simulink model "Hardmon"  (R2025b)
settings: Solver=ode8  StartTime=0.0  StopTime=10  FixedStep=0.0001  RelTol=1e-3
undefined symbols (not defined in the file): BMS_Contactor_Command
settings Model: DataDictionary=rev3_data.sldd  Creator=heyka  LastModifiedBy=diego
settings DataIOCC: ExternalInput=test_temp.getElement('Temp 1'),test_temp.getElement('Temp 2')  LoadExternalInput=on
settings OptimizationCC: DefaultParameterBehavior=Inlined  EnhancedBackFolding=on  PassReuseOutputArgsThreshold=0.0  ZeroExternalMemoryAtStartup=off  ZeroInternalMemoryAtStartup=off  OptimizeBlockOrder=speed  DifferentSizesBufferReuse=on  OptimizationCustomize=off
settings DebuggingCC: SolverPrmCheckMsg=warning  ParameterTunabilityLossMsg=error  StateNameClashWarn=warning
settings HardwareCC: ProdBitPerInt=16.0  ProdBitPerPointer=16.0  ProdBitPerSizeT=16.0  ProdBitPerPtrDiffT=16.0  ProdLargestAtomicFloat=None  ProdWordSize=16.0  ProdHWDeviceType=STMicroelectronics->ST10/Super10
settings SFSimCC: MATLABDynamicMemAlloc=off  SimTargetLang=C++  SimDLTargetLibrary=mkl-dnn
settings RTWCC: GenCodeOnly=on  Toolchain=MinGW64 | gmake (64-bit Windows)  BuildConfiguration=Faster Runs  TargetLang=C++  GPUComputeCapability=3.5
settings CodeAppCC: ForceParamTrailComments=on  OperatorAnnotations=on  StateflowObjectComments=on
settings GRTTargetCC: TargetLangStandard=C++11 (ISO)  CodeInterfacePackaging=C++ class  SubcomponentCodeInterfacePackaging=C++ class

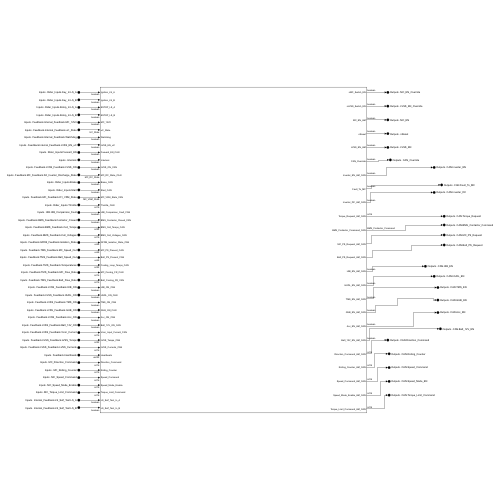
[thumbnail: Simulink's stored preview of the top-level diagram]
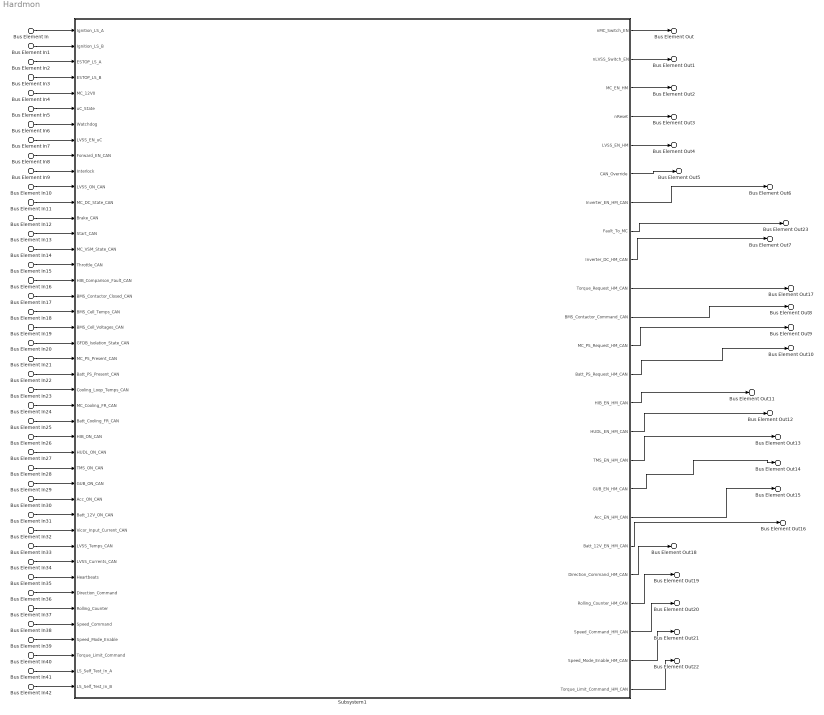
== system Hardmon ==
  Bus Element In2 : Inport  PortName=Inputs  Element=Rider_Inputs.Estop_In.LS_A
  Bus Element In3 : Inport  PortName=Inputs  Element=Rider_Inputs.Estop_In.LS_B
  Bus Element In1 : Inport  PortName=Inputs  Element=Rider_Inputs.Key_In.LS_B
  Bus Element In : Inport  PortName=Inputs  Element=Rider_Inputs.Key_In.LS_A
  Bus Element In8 : Inport  PortName=Inputs  Element=Rider_Inputs.Forward_EN
  Bus Element In12 : Inport  PortName=Inputs  Element=Rider_Inputs.Brake
  Bus Element In13 : Inport  PortName=Inputs  Element=Rider_Inputs.Start
  Bus Element In15 : Inport  PortName=Inputs  Element=Rider_Inputs.Throttle
  Bus Element In4 : Inport  PortName=Inputs  Element=Feedback.Internal_Feedback.MC_12V0
  Bus Element In5 : Inport  PortName=Inputs  Element=Feedback.Internal_Feedback.uC_State
  Bus Element In6 : Inport  PortName=Inputs  Element=Feedback.Internal_Feedback.Watchdog
  Bus Element In7 : Inport  PortName=Inputs  Element=Feedback.Internal_Feedback.LVSS_EN_uC
  Bus Element In10 : Inport  PortName=Inputs  Element=Feedback.LVSS_Feedback.LVSS_ON
  Bus Element In26 : Inport  PortName=Inputs  Element=Feedback.LVSS_Feedback.HIB_ON
  Bus Element In27 : Inport  PortName=Inputs  Element=Feedback.LVSS_Feedback.HUDL_ON
  Bus Element In28 : Inport  PortName=Inputs  Element=Feedback.LVSS_Feedback.TMS_ON
  Bus Element In29 : Inport  PortName=Inputs  Element=Feedback.LVSS_Feedback.GUB_ON
  Bus Element In30 : Inport  PortName=Inputs  Element=Feedback.LVSS_Feedback.Acc_ON
  Bus Element In31 : Inport  PortName=Inputs  Element=Feedback.LVSS_Feedback.Batt_12V_ON
  Bus Element In32 : Inport  PortName=Inputs  Element=Feedback.LVSS_Feedback.Vicor_Current
  Bus Element In33 : Inport  PortName=Inputs  Element=Feedback.LVSS_Feedback.LVSS_Temps
  Bus Element In34 : Inport  PortName=Inputs  Element=Feedback.LVSS_Feedback.LVSS_Currents
  Bus Element In11 : Inport  PortName=Inputs  Element=Feedback.MC_Feedback.D4_Inverter_Discharge_State
  Bus Element In14 : Inport  PortName=Inputs  Element=Feedback.MC_Feedback.D1_VSM_State
  Bus Element In17 : Inport  PortName=Inputs  Element=Feedback.BMS_Feedback.Contactor_Closed
  Bus Element In18 : Inport  PortName=Inputs  Element=Feedback.BMS_Feedback.Cell_Temps
  Bus Element In19 : Inport  PortName=Inputs  Element=Feedback.BMS_Feedback.Cell_Voltages
  Bus Element In20 : Inport  PortName=Inputs  Element=Feedback.GFDB_Feedback.Isolation_State
  Bus Element In21 : Inport  PortName=Inputs  Element=Feedback.TMS_Feedback.MC_Speed_Out
  Bus Element In22 : Inport  PortName=Inputs  Element=Feedback.TMS_Feedback.Batt_Speed_Out
  Bus Element In23 : Inport  PortName=Inputs  Element=Feedback.TMS_Feedback.Temperatures
  Bus Element In24 : Inport  PortName=Inputs  Element=Feedback.TMS_Feedback.MC_Flow_Rate
  Bus Element In25 : Inport  PortName=Inputs  Element=Feedback.TMS_Feedback.Batt_Flow_Rate
  Bus Element In35 : Inport  PortName=Inputs  Element=Feedback.Heartbeats
  Bus Element In9 : Inport  PortName=Inputs  Element=Interlock
  Bus Element In16 : Inport  PortName=Inputs  Element=HIB.HIB_Comparison_Fault
  Bus Element In36 : Inport  PortName=Inputs  Element=MC_Direction_Command
  Bus Element In37 : Inport  PortName=Inputs  Element=MC_Rolling_Counter
  Bus Element In38 : Inport  PortName=Inputs  Element=MC_Speed_Command
  Bus Element In39 : Inport  PortName=Inputs  Element=MC_Speed_Mode_Enable
  Bus Element In40 : Inport  PortName=Inputs  Element=MC_Torque_Limit_Command
  Bus Element In41 : Inport  PortName=Inputs  Element=Internal_Feedback.LS_Self_Test.LS_A
  Bus Element In42 : Inport  PortName=Inputs  Element=Internal_Feedback.LS_Self_Test.LS_B
  Subsystem1 : Subsystem
  Bus Element Out : Outport  PortName=Outputs  Element=MC_EN_Override
  Bus Element Out1 : Outport  PortName=Outputs  Element=LVSS_EN_Override
  Bus Element Out2 : Outport  PortName=Outputs  Element=MC_EN
  Bus Element Out3 : Outport  PortName=Outputs  Element=nReset
  Bus Element Out4 : Outport  PortName=Outputs  Element=LVSS_EN
  Bus Element Out5 : Outport  PortName=Outputs  Element=CAN_Override
  Bus Element Out6 : Outport  PortName=Outputs  Element=CAN.Inverter_EN
  Bus Element Out23 : Outport  PortName=Outputs  Element=CAN.Fault_To_MC
  Bus Element Out7 : Outport  PortName=Outputs  Element=CAN.Inverter_DC
  Bus Element Out17 : Outport  PortName=Outputs  Element=CAN.Torque_Request
  Bus Element Out8 : Outport  PortName=Outputs  Element=CAN.BMS_Contactor_Command
  Bus Element Out9 : Outport  PortName=Outputs  Element=CAN.MC_PS_Request
  Bus Element Out10 : Outport  PortName=Outputs  Element=CAN.Batt_PS_Request
  Bus Element Out11 : Outport  PortName=Outputs  Element=CAN.HIB_EN
  Bus Element Out12 : Outport  PortName=Outputs  Element=CAN.HUDL_EN
  Bus Element Out13 : Outport  PortName=Outputs  Element=CAN.TMS_EN
  Bus Element Out14 : Outport  PortName=Outputs  Element=CAN.GUB_EN
  Bus Element Out15 : Outport  PortName=Outputs  Element=CAN.Acc_EN
  Bus Element Out16 : Outport  PortName=Outputs  Element=CAN.Batt_12V_EN
  Bus Element Out18 : Outport  PortName=Outputs  Element=CAN.Direction_Command
  Bus Element Out19 : Outport  PortName=Outputs  Element=CAN.Rolling_Counter
  Bus Element Out20 : Outport  PortName=Outputs  Element=CAN.Speed_Command
  Bus Element Out21 : Outport  PortName=Outputs  Element=CAN.Speed_Mode_EN
  Bus Element Out22 : Outport  PortName=Outputs  Element=CAN.Torque_Limit_Command
  wires:
  Bus Element In/1 -> Subsystem1/1(Ignition_LS_A)
  Bus Element In1/1 -> Subsystem1/2(Ignition_LS_B)
  Bus Element In2/1 -> Subsystem1/3(ESTOP_LS_A)
  Bus Element In3/1 -> Subsystem1/4(ESTOP_LS_B)
  Bus Element In4/1 -> Subsystem1/5(MC_12V0)
  Bus Element In5/1 -> Subsystem1/6(uC_State)
  Bus Element In6/1 -> Subsystem1/7(Watchdog)
  Bus Element In7/1 -> Subsystem1/8(LVSS_EN_uC)
  Bus Element In8/1 -> Subsystem1/9(Forward_EN_CAN)
  Bus Element In9/1 -> Subsystem1/10(Interlock)
  Bus Element In10/1 -> Subsystem1/11(LVSS_ON_CAN)
  Bus Element In11/1 -> Subsystem1/12(MC_DC_State_CAN)
  Bus Element In12/1 -> Subsystem1/13(Brake_CAN)
  Bus Element In13/1 -> Subsystem1/14(Start_CAN)
  Bus Element In14/1 -> Subsystem1/15(MC_VSM_State_CAN)
  Bus Element In15/1 -> Subsystem1/16(Throttle_CAN)
  Bus Element In16/1 -> Subsystem1/17(HIB_Comparison_Fault_CAN)
  Bus Element In17/1 -> Subsystem1/18(BMS_Contactor_Closed_CAN)
  Bus Element In18/1 -> Subsystem1/19(BMS_Cell_Temps_CAN)
  Bus Element In19/1 -> Subsystem1/20(BMS_Cell_Voltages_CAN)
  Bus Element In20/1 -> Subsystem1/21(GFDB_Isolation_State_CAN)
  Bus Element In21/1 -> Subsystem1/22(MC_PS_Present_CAN)
  Bus Element In22/1 -> Subsystem1/23(Batt_PS_Present_CAN)
  Bus Element In23/1 -> Subsystem1/24(Cooling_Loop_Temps_CAN)
  Bus Element In24/1 -> Subsystem1/25(MC_Cooling_FR_CAN)
  Bus Element In25/1 -> Subsystem1/26(Batt_Cooling_FR_CAN)
  Bus Element In26/1 -> Subsystem1/27(HIB_ON_CAN)
  Bus Element In27/1 -> Subsystem1/28(HUDL_ON_CAN)
  Bus Element In28/1 -> Subsystem1/29(TMS_ON_CAN)
  Bus Element In29/1 -> Subsystem1/30(GUB_ON_CAN)
  Bus Element In30/1 -> Subsystem1/31(Acc_ON_CAN)
  Bus Element In31/1 -> Subsystem1/32(Batt_12V_ON_CAN)
  Bus Element In32/1 -> Subsystem1/33(Vicor_Input_Current_CAN)
  Bus Element In33/1 -> Subsystem1/34(LVSS_Temps_CAN)
  Bus Element In34/1 -> Subsystem1/35(LVSS_Currents_CAN)
  Bus Element In35/1 -> Subsystem1/36(Heartbeats)
  Bus Element In36/1 -> Subsystem1/37(Direction_Command)
  Bus Element In37/1 -> Subsystem1/38(Rolling_Counter)
  Bus Element In38/1 -> Subsystem1/39(Speed_Command)
  Bus Element In39/1 -> Subsystem1/40(Speed_Mode_Enable)
  Bus Element In40/1 -> Subsystem1/41(Torque_Limit_Command)
  Bus Element In41/1 -> Subsystem1/42(LS_Self_Test_In_A)
  Bus Element In42/1 -> Subsystem1/43(LS_Self_Test_In_B)
  Subsystem1/1(nMC_Switch_EN) -> Bus Element Out/1
  Subsystem1/2(nLVSS_Switch_EN) -> Bus Element Out1/1
  Subsystem1/3(MC_EN_HM) -> Bus Element Out2/1
  Subsystem1/4(nReset) -> Bus Element Out3/1
  Subsystem1/5(LVSS_EN_HM) -> Bus Element Out4/1
  Subsystem1/6(CAN_Override) -> Bus Element Out5/1
  Subsystem1/7(Inverter_EN_HM_CAN) -> Bus Element Out6/1
  Subsystem1/9(Inverter_DC_HM_CAN) -> Bus Element Out7/1
  Subsystem1/11(BMS_Contactor_Command_CAN) -> Bus Element Out8/1
  Subsystem1/12(MC_PS_Request_HM_CAN) -> Bus Element Out9/1
  Subsystem1/13(Batt_PS_Request_HM_CAN) -> Bus Element Out10/1
  Subsystem1/14(HIB_EN_HM_CAN) -> Bus Element Out11/1
  Subsystem1/15(HUDL_EN_HM_CAN) -> Bus Element Out12/1
  Subsystem1/16(TMS_EN_HM_CAN) -> Bus Element Out13/1
  Subsystem1/17(GUB_EN_HM_CAN) -> Bus Element Out14/1
  Subsystem1/18(Acc_EN_HM_CAN) -> Bus Element Out15/1
  Subsystem1/19(Batt_12V_EN_HM_CAN) -> Bus Element Out16/1
  Subsystem1/10(Torque_Request_HM_CAN) -> Bus Element Out17/1
  Subsystem1/20(Direction_Command_HM_CAN) -> Bus Element Out18/1
  Subsystem1/21(Rolling_Counter_HM_CAN) -> Bus Element Out19/1
  Subsystem1/22(Speed_Command_HM_CAN) -> Bus Element Out20/1
  Subsystem1/23(Speed_Mode_Enable_HM_CAN) -> Bus Element Out21/1
  Subsystem1/24(Torque_Limit_Command_HM_CAN) -> Bus Element Out22/1
  Subsystem1/8(Fault_To_MC) -> Bus Element Out23/1

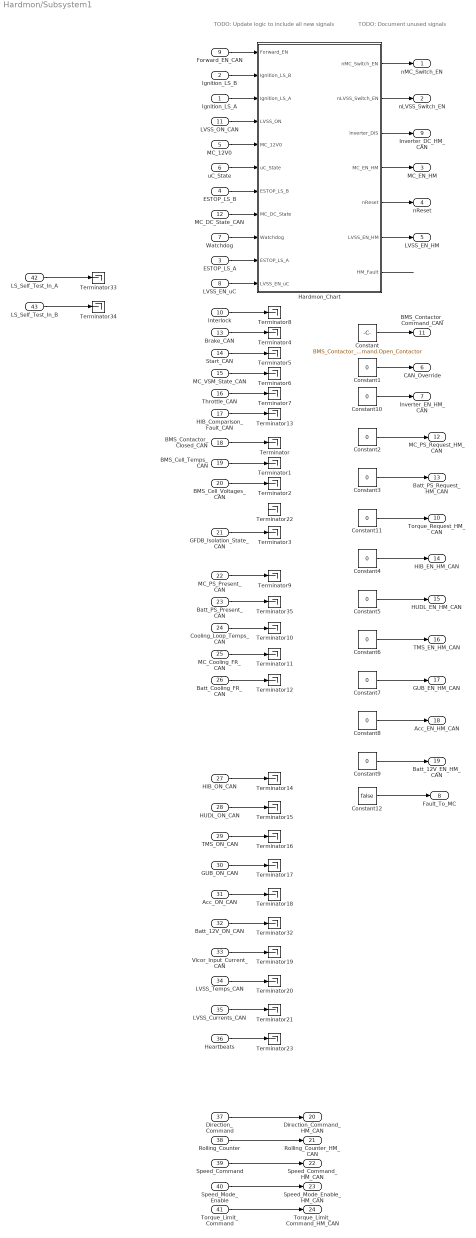
== system Hardmon/Subsystem1 ==
  note: TODO: Update logic to include all new signals
  note: TODO: Document unused signals
  Ignition_LS_A : Inport  OutDataTypeStr=boolean
  Ignition_LS_B : Inport  Port=2  OutDataTypeStr=boolean
  ESTOP_LS_A : Inport  Port=3  OutDataTypeStr=boolean
  ESTOP_LS_B : Inport  Port=4  OutDataTypeStr=boolean
  MC_12V0 : Inport  Port=5  OutDataTypeStr=boolean
  uC_State : Inport  Port=6  OutDataTypeStr=Enum: UC_State
  Watchdog : Inport  Port=7  OutDataTypeStr=boolean
  LVSS_EN_uC : Inport  Port=8  OutDataTypeStr=boolean
  Forward_EN_CAN : Inport  Port=9  OutDataTypeStr=boolean
  Interlock : Inport  Port=10  OutDataTypeStr=boolean
  LVSS_ON_CAN : Inport  Port=11  OutDataTypeStr=boolean
  MC_DC_State_CAN : Inport  Port=12  OutDataTypeStr=Enum: MC_DC_State
  Brake_CAN : Inport  Port=13  OutDataTypeStr=boolean
  Start_CAN : Inport  Port=14  OutDataTypeStr=boolean
  MC_VSM_State_CAN : Inport  Port=15  OutDataTypeStr=Enum: MC_VSM_State
  Throttle_CAN : Inport  Port=16  OutDataTypeStr=int16
  HIB_Comparison_Fault_CAN : Inport  Port=17  OutDataTypeStr=boolean
  BMS_Contactor_Closed_CAN : Inport  Port=18  OutDataTypeStr=boolean
  BMS_Cell_Temps_CAN : Inport  Port=19  OutDataTypeStr=int32  PortDimensions=[1,45]
  BMS_Cell_Voltages_CAN : Inport  Port=20  OutDataTypeStr=int16  PortDimensions=[1,100]
  GFDB_Isolation_State_CAN : Inport  Port=21  OutDataTypeStr=uint8
  MC_PS_Present_CAN : Inport  Port=22  OutDataTypeStr=uint8
  Batt_PS_Present_CAN : Inport  Port=23  OutDataTypeStr=uint8
  Cooling_Loop_Temps_CAN : Inport  Port=24  OutDataTypeStr=int32  PortDimensions=[1,5]
  MC_Cooling_FR_CAN : Inport  Port=25  OutDataTypeStr=int16
  Batt_Cooling_FR_CAN : Inport  Port=26  OutDataTypeStr=int16
  HIB_ON_CAN : Inport  Port=27  OutDataTypeStr=boolean
  HUDL_ON_CAN : Inport  Port=28  OutDataTypeStr=boolean
  TMS_ON_CAN : Inport  Port=29  OutDataTypeStr=boolean
  GUB_ON_CAN : Inport  Port=30  OutDataTypeStr=boolean
  Acc_ON_CAN : Inport  Port=31  OutDataTypeStr=boolean
  Batt_12V_ON_CAN : Inport  Port=32  OutDataTypeStr=boolean
  Vicor_Input_Current_CAN : Inport  Port=33  OutDataTypeStr=int16
  LVSS_Temps_CAN : Inport  Port=34  OutDataTypeStr=int32  PortDimensions=[1,6]
  LVSS_Currents_CAN : Inport  Port=35  OutDataTypeStr=int16  PortDimensions=[1,6]
  Heartbeats : Inport  Port=36  OutDataTypeStr=uint32  PortDimensions=[1,5]
  Direction_Command : Inport  Port=37  OutDataTypeStr=int16
  Rolling_Counter : Inport  Port=38  OutDataTypeStr=int16
  Speed_Command : Inport  Port=39  OutDataTypeStr=int16
  Speed_Mode_Enable : Inport  Port=40  OutDataTypeStr=int16
  Torque_Limit_Command : Inport  Port=41  OutDataTypeStr=int16
  LS_Self_Test_In_A : Inport  Port=42  OutDataTypeStr=boolean
  LS_Self_Test_In_B : Inport  Port=43  OutDataTypeStr=boolean
  Constant : Constant  Value=BMS_Contactor_Command.Open_Contactor  OutDataTypeStr=Enum: BMS_Contactor_Command
  Constant{1,4..10} (8 alike) : Constant  Value=0  OutDataTypeStr=boolean
  Constant11 : Constant  Value=0  OutDataTypeStr=int16
  Constant12 : Constant  Value=false  OutDataTypeStr=boolean
  Constant2 : Constant  Value=0  OutDataTypeStr=uint8
  Constant3 : Constant  Value=0  OutDataTypeStr=uint8
  Hardmon_Chart : Stateflow chart  TreatAsAtomicUnit=on
      settings: PortSchema="{\"entries\":[{\"content\":{\"sides\":[{\"content\":{\"connectorIds\":[\"In1\",\"In2\",\"In3\",\"In4\",\"In5\",\"In6\",\"In7\",\"In8\",\"In9\",\"In10\",\"In11\"]},\"type\":\"ConnectorPlacement.EquallySpacedRectSide\",\"uuid\":\"6d1a41ef-67e8-41d6-9adb-1761831f6d0e\"},{\"content\":{\"connectorIds\":[\"Out1\",\"Out7\",\"Out2\",\"Out3\",\"Out4\",\"Out5\",\"Out6\"],\"side\":\"RIGHT\"},\"type\":\"ConnectorPlacement.EquallySpacedRectSide\",\"uuid\":\"1c1f5b1f-9a19-48ee-ac61-8a13c1cfd4a8\"},{\"content\":{\"side\":\"TOP\"},\"type\":\"ConnectorPlacement.EquallySpacedRectSide\",\"uuid\":\"7f8ec887-50f7-4fb3-9eed-5aef04cf2afb\"}]},\"type\":\"ConnectorPlacement.EquallySpacedConnector\",\"uuid\":\"822c8876-1e52-4482-83f3-7114ae95ed93\"}],\"packageUris\":[\"http://schema.mathworks.com/mf0/Connector/R2020b\"],\"version\":\"1.0\"}"
  Terminator{,1..23,32..35} (28 alike) : Terminator
  nMC_Switch_EN : Outport  OutDataTypeStr=boolean
  nLVSS_Switch_EN : Outport  Port=2  OutDataTypeStr=boolean
  MC_EN_HM : Outport  Port=3  OutDataTypeStr=boolean
  nReset : Outport  Port=4  OutDataTypeStr=boolean
  LVSS_EN_HM : Outport  Port=5  OutDataTypeStr=boolean
  CAN_Override : Outport  Port=6  OutDataTypeStr=boolean
  Inverter_EN_HM_CAN : Outport  Port=7  OutDataTypeStr=boolean
  Fault_To_MC : Outport  Port=8  OutDataTypeStr=boolean
  Inverter_DC_HM_CAN : Outport  Port=9  OutDataTypeStr=boolean
  Torque_Request_HM_CAN : Outport  Port=10  OutDataTypeStr=int16
  BMS_Contactor_Command_CAN : Outport  Port=11  OutDataTypeStr=Enum: BMS_Contactor_Command
  MC_PS_Request_HM_CAN : Outport  Port=12
  Batt_PS_Request_HM_CAN : Outport  Port=13
  HIB_EN_HM_CAN : Outport  Port=14  OutDataTypeStr=boolean
  HUDL_EN_HM_CAN : Outport  Port=15  OutDataTypeStr=boolean
  TMS_EN_HM_CAN : Outport  Port=16  OutDataTypeStr=boolean
  GUB_EN_HM_CAN : Outport  Port=17  OutDataTypeStr=boolean
  Acc_EN_HM_CAN : Outport  Port=18  OutDataTypeStr=boolean
  Batt_12V_EN_HM_CAN : Outport  Port=19  OutDataTypeStr=boolean
  Direction_Command_HM_CAN : Outport  Port=20  OutDataTypeStr=int16
  Rolling_Counter_HM_CAN : Outport  Port=21  OutDataTypeStr=int16
  Speed_Command_HM_CAN : Outport  Port=22  OutDataTypeStr=int16
  Speed_Mode_Enable_HM_CAN : Outport  Port=23  OutDataTypeStr=int16
  Torque_Limit_Command_HM_CAN : Outport  Port=24  OutDataTypeStr=int16
  wires:
  Vicor_Input_Current_CAN/1 -> Terminator19/1
  LVSS_Temps_CAN/1 -> Terminator20/1
  MC_PS_Present_CAN/1 -> Terminator9/1
  Torque_Limit_Command/1 -> Torque_Limit_Command_HM_CAN/1
  Heartbeats/1 -> Terminator23/1
  Throttle_CAN/1 -> Terminator7/1
  ? -> Terminator22/1
  BMS_Cell_Temps_CAN/1 -> Terminator1/1
  Hardmon_Chart/1(nMC_Switch_EN) -> nMC_Switch_EN/1
  HIB_ON_CAN/1 -> Terminator14/1
  Constant9/1 -> Batt_12V_EN_HM_CAN/1
  LVSS_Currents_CAN/1 -> Terminator21/1
  Constant11/1 -> Torque_Request_HM_CAN/1
  Rolling_Counter/1 -> Rolling_Counter_HM_CAN/1
  BMS_Cell_Voltages_CAN/1 -> Terminator2/1
  MC_12V0/1 -> Hardmon_Chart/5(MC_12V0)
  GUB_ON_CAN/1 -> Terminator17/1
  Direction_Command/1 -> Direction_Command_HM_CAN/1
  HUDL_ON_CAN/1 -> Terminator15/1
  MC_DC_State_CAN/1 -> Hardmon_Chart/8(MC_DC_State)
  Hardmon_Chart/4(nReset) -> nReset/1
  LVSS_EN_uC/1 -> Hardmon_Chart/11(LVSS_EN_uC)
  Constant7/1 -> GUB_EN_HM_CAN/1
  Constant10/1 -> Inverter_EN_HM_CAN/1
  LVSS_ON_CAN/1 -> Hardmon_Chart/4(LVSS_ON)
  Speed_Mode_Enable/1 -> Speed_Mode_Enable_HM_CAN/1
  Ignition_LS_A/1 -> Hardmon_Chart/3(Ignition_LS_A)
  MC_Cooling_FR_CAN/1 -> Terminator11/1
  ESTOP_LS_A/1 -> Hardmon_Chart/10(ESTOP_LS_A)
  Constant8/1 -> Acc_EN_HM_CAN/1
  ESTOP_LS_B/1 -> Hardmon_Chart/7(ESTOP_LS_B)
  MC_VSM_State_CAN/1 -> Terminator6/1
  Constant/1 -> BMS_Contactor_Command_CAN/1
  Batt_PS_Present_CAN/1 -> Terminator35/1
  Forward_EN_CAN/1 -> Hardmon_Chart/1(Forward_EN)
  TMS_ON_CAN/1 -> Terminator16/1
  Brake_CAN/1 -> Terminator4/1
  Batt_Cooling_FR_CAN/1 -> Terminator12/1
  HIB_Comparison_Fault_CAN/1 -> Terminator13/1
  BMS_Contactor_Closed_CAN/1 -> Terminator/1
  Constant6/1 -> TMS_EN_HM_CAN/1
  Constant4/1 -> HIB_EN_HM_CAN/1
  Hardmon_Chart/7(nLVSS_Switch_EN) -> nLVSS_Switch_EN/1
  Hardmon_Chart/2(Inverter_DIS) -> Inverter_DC_HM_CAN/1
  LS_Self_Test_In_A/1 -> Terminator33/1
  Batt_12V_ON_CAN/1 -> Terminator32/1
  Constant3/1 -> Batt_PS_Request_HM_CAN/1
  Constant2/1 -> MC_PS_Request_HM_CAN/1
  Cooling_Loop_Temps_CAN/1 -> Terminator10/1
  GFDB_Isolation_State_CAN/1 -> Terminator3/1
  Speed_Command/1 -> Speed_Command_HM_CAN/1
  Start_CAN/1 -> Terminator5/1
  LS_Self_Test_In_B/1 -> Terminator34/1
  Hardmon_Chart/5(LVSS_EN_HM) -> LVSS_EN_HM/1
  Hardmon_Chart/3(MC_EN_HM) -> MC_EN_HM/1
  Constant5/1 -> HUDL_EN_HM_CAN/1
  Ignition_LS_B/1 -> Hardmon_Chart/2(Ignition_LS_B)
  Hardmon_Chart/6(HM_Fault) -> ?
  uC_State/1 -> Hardmon_Chart/6(uC_State)
  Acc_ON_CAN/1 -> Terminator18/1
  Watchdog/1 -> Hardmon_Chart/9(Watchdog)
  Constant1/1 -> CAN_Override/1
  Interlock/1 -> Terminator8/1
  Constant12/1 -> Fault_To_MC/1

== stateflow chart Hardmon/Subsystem1/Hardmon_Chart ==
  note: General Notes:
      | - LVSS_EN_HM = LVSS_EN_uC is used to ensure that if the HardMon triggers
      | - No transitions occur when the uC_State is 6 or 7 to ensure that nothing tranistions when the motor controller is already discharging
  state Normal_Operation
    state ESTOP_Checking [parallel]
      settings: executionOrder=1
      state count
        entry:
        ESTOP_Counter = ESTOP_Counter + 1;
      state ESTOP_Inactive
        entry:
        HM_Fault = false;
        ESTOP_Counter = 0;
        nMC_Switch_EN = false;
        nLVSS_Switch_EN = false;
        LVSS_EN_HM = LVSS_EN_uC;
      (default) -> ESTOP_Inactive
      ESTOP_Inactive -> Normal_Operation.ESTOP_Checking.count : [ESTOP_LS_A == true && uC_State ~= UC_State.Fault && uC_State ~= UC_State.Estop ]
      Normal_Operation.ESTOP_Checking.count -> ESTOP_Inactive [order 2] : [ESTOP_LS_A == true || uC_State == UC_State.Fault || uC_State == UC_State.Estop ]
      Normal_Operation.ESTOP_Checking.count -> Normal_Operation.ESTOP_Checking.count [order 1] : after(0.1,sec)
    state Watchdog_Checking [parallel]
      settings: executionOrder=2
      state WD_Low
        entry:
        WD_Counter = 0;
        state Counting
          entry:
          WD_Counter = WD_Counter + 1;
        Normal_Operation.Watchdog_Checking.WD_Low.Counting -> Normal_Operation.Watchdog_Checking.WD_Low.Counting [order 2] : after(0.5, sec)
      state WD_High
        entry:
        WD_Counter = 0;
        state Counting
          entry:
          WD_Counter = WD_Counter + 1;
        Normal_Operation.Watchdog_Checking.WD_High.Counting -> Normal_Operation.Watchdog_Checking.WD_High.Counting [order 2] : after(0.5, sec)
      (default) -> WD_Low
      Normal_Operation.Watchdog_Checking.WD_Low.Counting -> WD_High [order 1] : [Watchdog == true]
      Normal_Operation.Watchdog_Checking.WD_High.Counting -> WD_Low [order 1] : [Watchdog == false]
    state Invalid_State_Checking [parallel]
      settings: executionOrder=3
      state count
        entry:
        Invalid_State_Counter = Invalid_State_Counter + 1;
      state Invalid_State_Inactive
        entry:
        HM_Fault = false;
        Invalid_State_Counter = 0;
        nMC_Switch_EN = false;
        nLVSS_Switch_EN = false;
        LVSS_EN_HM = LVSS_EN_uC;
      (default) -> Normal_Operation.Invalid_State_Checking.Invalid_State_Inactive
      Normal_Operation.Invalid_State_Checking.Invalid_State_Inactive -> Normal_Operation.Invalid_State_Checking.count : [(Forward_EN ~= true || Ignition_LS_A ~= true) && uC_State == UC_State.MC_Active]
      Normal_Operation.Invalid_State_Checking.count -> Normal_Operation.Invalid_State_Checking.Invalid_State_Inactive [order 2] : [~((Forward_EN ~= true || Ignition_LS_A ~= true) && uC_State == UC_State.MC_Active)]
      Normal_Operation.Invalid_State_Checking.count -> Normal_Operation.Invalid_State_Checking.count [order 1] : after(0.5,sec)
    state Ignition_Level_Checking [parallel]
      settings: executionOrder=4
      state count
        entry:
        Ignition_State_Counter = Ignition_State_Counter + 1;
      state Ignition_State_Inactive
        entry:
        HM_Fault = false;
        Ignition_State_Counter = 0;
        nMC_Switch_EN = false;
        nLVSS_Switch_EN = false;
        LVSS_EN_HM = LVSS_EN_uC;
      (default) -> Ignition_State_Inactive
      Ignition_State_Inactive -> Normal_Operation.Ignition_Level_Checking.count : [Ignition_LS_A ~= Ignition_LS_B  && uC_State ~= UC_State.Fault]
      Normal_Operation.Ignition_Level_Checking.count -> Ignition_State_Inactive [order 2] : [Ignition_LS_A == Ignition_LS_B  || uC_State == UC_State.Fault ]
      Normal_Operation.Ignition_Level_Checking.count -> Normal_Operation.Ignition_Level_Checking.count [order 1] : after(0.5,sec)
    state ESTOP_Level_Checking [parallel]
      settings: executionOrder=5
      state count
        entry:
        ESTOP_State_Counter = ESTOP_State_Counter + 1;
      state ESTOP_State_Inactive
        entry:
        HM_Fault = false;
        ESTOP_State_Counter = 0;
        nMC_Switch_EN = false;
        nLVSS_Switch_EN = false;
        LVSS_EN_HM = LVSS_EN_uC;
      (default) -> ESTOP_State_Inactive
      ESTOP_State_Inactive -> Normal_Operation.ESTOP_Level_Checking.count : [ESTOP_LS_A ~= ESTOP_LS_B  && uC_State ~= UC_State.Fault ]
      Normal_Operation.ESTOP_Level_Checking.count -> ESTOP_State_Inactive [order 2] : [ESTOP_LS_A == ESTOP_LS_B  || uC_State == UC_State.Fault ]
      Normal_Operation.ESTOP_Level_Checking.count -> Normal_Operation.ESTOP_Level_Checking.count [order 1] : after(0.5,sec)
    state LVSS_Checking [parallel]
      settings: executionOrder=6
      state count
        entry:
        LVSS_Counter = LVSS_Counter + 1;
      state Invalid_State_Inactive
        entry:
        HM_Fault = false;
        LVSS_Counter = 0;
        nMC_Switch_EN = false;
        nLVSS_Switch_EN = false;
        LVSS_EN_HM = LVSS_EN_uC;
      (default) -> Normal_Operation.LVSS_Checking.Invalid_State_Inactive
      Normal_Operation.LVSS_Checking.Invalid_State_Inactive -> Normal_Operation.LVSS_Checking.count : [LVSS_ON ~= LVSS_EN_uC  && uC_State ~= UC_State.Fault ]
      Normal_Operation.LVSS_Checking.count -> Normal_Operation.LVSS_Checking.Invalid_State_Inactive [order 2] : [LVSS_ON == LVSS_EN_uC  || uC_State == UC_State.Fault ]
      Normal_Operation.LVSS_Checking.count -> Normal_Operation.LVSS_Checking.count [order 1] : after(0.5,sec)
  note: RESET
      | - Only occurs when the watchdog faults
      | - Ensure that the motor controller and lvss is correclty shutdown and holds the MCuC in the reset state
  note: ESTOP Checking:
      | - Checks for ESTOP being triggered but MCUC not entering ESTOP state
  state MC_RESET_INIT
    entry:
    nMC_Switch_EN = true;
    nLVSS_Switch_EN = true;
  state MC_DISCHARGE
    entry:
    HM_Fault = true;
    Inverter_DIS = true;
  note: Watchdog_Checking
      | - Checks that the MCuC is operational by requiring a constant watchdog gpio to be toggled by the MCuC
      | - Applies a hardware reset instead of triggering a fault
  note: Invalid State Checking
      | - Checks if the MCuC being in the active state is possible given the current inputs
      | - Only valid during the MCuC active state
  state MC_POWERDOWN
    entry:
    nReset = false;
    Inverter_DIS = false;
    MC_EN_HM = false;
  note: Ignition Level Checking
      | - Ensures that the ignition signal matches with both level shifters
  note: ESTOP Level Checking
      | - Ensures that the ESTOP signal matches with both level shifters
  note: LVSS Status Checking
      | - Ensures that the LVSS status matches the LVSS ON command
  state LVSS_Powerdown
    entry:
    LVSS_EN_HM = false;
  state Enter_Fault
    entry:
    nReset = true;
    HM_Fault = true;
    exit:
    nMC_Switch_EN = false;
    nLVSS_Switch_EN = false;
    nReset = false;
  note: Fault
      | - Normal fault handling, ensures the correct shutdown of motor controller and LVSS
  state MC_FAULT_INIT
    entry:
    nMC_Switch_EN = true;
    nLVSS_Switch_EN = true;
  state MC_DISCHARGE_FAULT
    entry:
    HM_Fault = true;
    Inverter_DIS = true;
  state MC_POWERDOWN1
    entry:
    HM_Fault  = true;
    Inverter_DIS = false;
    MC_EN_HM = false;
  state LVSS_Powerdown1
    entry:
    LVSS_EN_HM = false;
  state End_Powerdown
    entry:
    nMC_Switch_EN = false;
    nLVSS_Switch_EN = false;
    exit:
    HM_Fault = true;
  (default) -> Normal_Operation
  MC_RESET_INIT -> MC_DISCHARGE [order 1] : [uC_State ~= UC_State.MC_Off && uC_State ~= UC_State.Preset]
  Normal_Operation -> MC_RESET_INIT [order 1] : [WD_Counter >= 4 && uC_State ~= UC_State.Preset]
  MC_RESET_INIT -> MC_POWERDOWN [order 2] : [uC_State == UC_State.MC_Off || uC_State == UC_State.Preset]
  MC_DISCHARGE -> MC_POWERDOWN : [MC_DC_State == 4]
  MC_POWERDOWN -> LVSS_Powerdown : [MC_12V0 == false]
  LVSS_Powerdown -> Enter_Fault : [LVSS_ON == false]
  Enter_Fault -> Normal_Operation : [uC_State == 8]
  Normal_Operation -> MC_FAULT_INIT [order 2] : [Invalid_State_Counter >= 4 || Ignition_State_Counter >= 4 || LVSS_Counter >=4 || ESTOP_Counter >= 4 || ESTOP_State_Counter >= 4]
  MC_FAULT_INIT -> MC_DISCHARGE_FAULT [order 1] : [uC_State ~= UC_State.MC_Off && uC_State ~= UC_State.Preset]
  MC_FAULT_INIT -> MC_POWERDOWN1 [order 2] : [uC_State == UC_State.MC_Off || uC_State == UC_State.Preset]
  MC_DISCHARGE_FAULT -> MC_POWERDOWN1 : [MC_DC_State == 4]
  MC_POWERDOWN1 -> LVSS_Powerdown1 : [MC_12V0 == false]
  LVSS_Powerdown1 -> End_Powerdown : [LVSS_ON == false]
  End_Powerdown -> Normal_Operation : [uC_State == 6]
  data: WD_Counter local; Forward_EN input; Ignition_LS_B input; Ignition_LS_A input; LVSS_ON input; MC_12V0 input; uC_State input; nMC_Switch_EN output; Inverter_DIS output; MC_EN_HM output; nReset output =true; ESTOP_State_Counter local; Ignition_State_Counter local; Invalid_State_Counter local; LVSS_Counter local; LVSS_EN_HM output; ESTOP_LS_B input; MC_DC_State input; Watchdog input; ESTOP_Counter local; ESTOP_LS_A input =0; HM_Fault output; LVSS_EN_uC input; nLVSS_Switch_EN output
